simulink model "BattMPCv1"  (R2022b)
settings: Solver=VariableStepAuto  StartTime=0.0  StopTime=10.0  RelTol=1e-3
undefined symbols (not defined in the file): param
libraries: simulink x2, SOCMPC x1
settings Model: Creator=user  LastModifiedBy=user

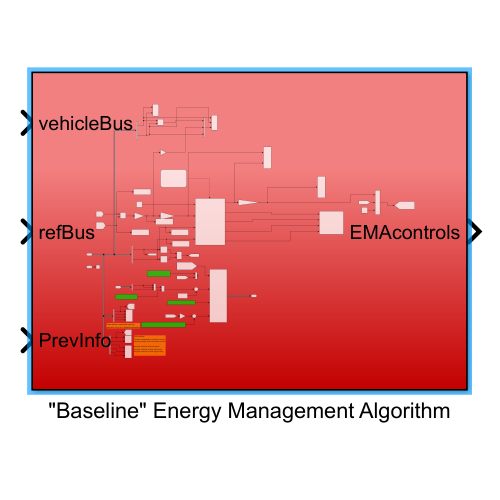
[thumbnail: Simulink's stored preview of the top-level diagram]
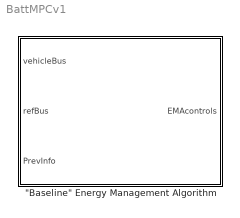
== system BattMPCv1 ==
  "\"Baseline\" Energy Management Algorithm" : Subsystem

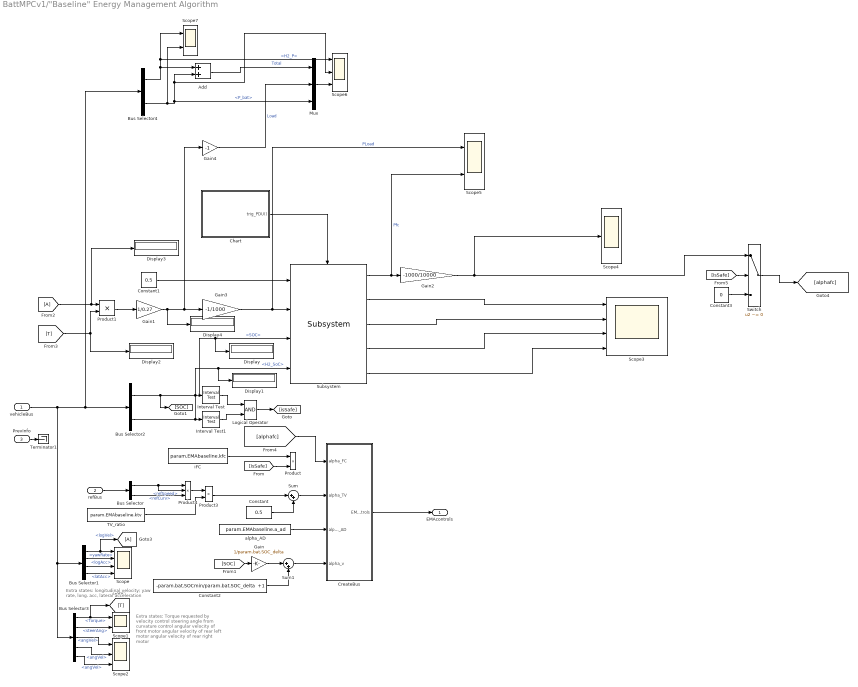
== system BattMPCv1/"Baseline" Energy Management Algorithm ==
  note: Extra states: longitudinal velocity;
      | yaw rate, long. acc, lateral acceleration
  note: Extra states:
      | Torque requested by velocity control
      | steering angle from curvature control
      |
      | angular velocity of front motor
      | angular velocity of rear left motor
      | angular velocity of rear right motor
  vehicleBus : Inport
  refBus : Inport  Port=2
  PrevInfo : Inport  Port=3
  Add : Sum
  Bus Selector : BusSelector  OutputSignals=refSpeed,refCurv
  Bus Selector1 : BusSelector  OutputSignals=chassisBus.logVel,chassisBus.yawRate,chassisBus.logAcc,chassisBus.latAcc
  Bus Selector2 : BusSelector  OutputSignals=batteryBus.SOC,rexBus.H2_SoC
  Bus Selector3 : BusSelector  OutputSignals=chassisControlBus.Torque,chassisControlBus.steerAng,electricMotorBusFM.angVel,electricMotorBusRL.angVel,electricMotorBusRR.angVel
  Bus Selector4 : BusSelector  OutputSignals=rexBus.H2_P,batteryBus.P_bat
  Chart : Stateflow chart  TreatAsAtomicUnit=on  SystemSampleTime=0.01
  Constant : Constant  Value=0.5
  Constant1 : Constant  Value=0.5
  Constant2 : Constant  Value="-param.bat.SOCmin/param.bat.SOC_delta  +1"
  Constant3 : Constant  Value=0
  CreateBus : Subsystem
  Display{,1..4} (5 alike) : Display
  From2 : From
  Gain : Gain  Gain=1/param.bat.SOC_delta
  Gain1 : Gain  Gain=1/0.27
  Gain2 : Gain  Gain=-1000/10000
  Gain3 : Gain  Gain=-1/1000
  Gain4 : Gain  Gain=-1
  Goto3 : Goto
  Interval Test : simulink/Logic and Bit Operations/Interval Test  IntervalClosedRight=on  uplimit=param.bat.SOCmax  IntervalClosedLeft=on  lowlimit=param.bat.SOCmin  OutDataTypeStr=boolean
  Interval Test1 : simulink/Logic and Bit Operations/Interval Test  IntervalClosedRight=on  uplimit=param.fuelcell.SOCmax  IntervalClosedLeft=on  lowlimit=param.fuelcell.SOCmin  OutDataTypeStr=boolean
  Logical Operator : Logic  AllPortsSameDT=off  OutDataTypeStr=boolean
  Mux : Mux  Inputs=3
  Product : Product
  Product1 : Product
  Product3 : Product
  Product4 : Product  Inputs=3
  Scope : Scope  NumInputPorts=4
  Scope1 : Scope  NumInputPorts=2
  Scope2 : Scope  NumInputPorts=3
  Scope3 : Scope  NumInputPorts=4
  Scope4 : Scope
  Scope5 : Scope  NumInputPorts=2
  Scope6 : Scope  NumInputPorts=3
  Scope7 : Scope  NumInputPorts=2
  Subsystem : SOCMPC/Subsystem  SystemSampleTime=-1  VariantActivationTime=update diagram  Latency=0  AutoFrameSizeCalculation=off
      link override Constrained: Gain=1
      link override Not Constrained: Gain=1
  Sum : Sum  Inputs=|++
  Sum1 : Sum  Inputs=|++
  Switch : Switch  Criteria=u2 ~= 0  SaturateOnIntegerOverflow=off  InputSameDT=off
  TV_ratio : Constant  Value=param.EMAbaseline.ktv
  Terminator1 : Terminator
  alpha_AD : Constant  Value=param.EMAbaseline.a_ad
  iFC : Constant  Value=param.EMAbaseline.kfc
  EMAcontrols : Outport
  wires:
  vehicleBus/1 -> Bus Selector4/1, Bus Selector2/1, Bus Selector3/1, Bus Selector1/1
  iFC/1 -> Product/1
  Bus Selector2/2 -> Display1/1, Subsystem/4, Interval Test1/1  "<H2_SoC>"
  Bus Selector2/1 -> [SOC], Display/1, Subsystem/3, Interval Test/1  "<SOC>"
  Interval Test/1 -> Logical Operator/1
  Interval Test1/1 -> Logical Operator/2
  CreateBus/1(EMAcontrols) -> EMAcontrols/1
  Logical Operator/1 -> [isSafe]
  [isSafe] -> Product/2
  TV_ratio/1 -> Product3/2
  Product4/1 -> Product3/1
  refBus/1 -> Bus Selector/1
  Bus Selector/2 -> Product4/3  "<refCurv>"
  Bus Selector/1 -> Product4/2, Product4/1  "<refSpeed>"
  Constant/1 -> Sum/2
  Product3/1 -> Sum/1
  [SOC] -> Gain/1
  Gain/1 -> Sum1/1
  Constant2/1 -> Sum1/2
  PrevInfo/1 -> Terminator1/1
  Sum/1 -> CreateBus/2(alpha_TV)
  alpha_AD/1 -> CreateBus/3(alpha_AD)
  Sum1/1 -> CreateBus/4(alpha_v)
  Bus Selector1/1 -> Goto3/1, Scope/1  "<logVel>"
  Bus Selector1/2 -> Scope/2  "<yawRate>"
  Bus Selector1/3 -> Scope/3  "<logAcc>"
  Bus Selector1/4 -> Scope/4  "<latAcc>"
  Bus Selector3/1 -> [T], Scope1/1  "<Torque>"
  Bus Selector3/2 -> Scope1/2  "<steerAng>"
  Bus Selector3/3 -> Scope2/1  "<angVel>"
  Bus Selector3/4 -> Scope2/2  "<angVel>"
  Bus Selector3/5 -> Scope2/3  "<angVel>"
  Constant1/1 -> Subsystem/1
  From2/1 -> Display3/1, Product1/1
  [T] -> Product1/2, Display2/1
  Product1/1 -> Gain1/1
  Gain1/1 -> Display4/1, Gain4/1, Gain3/1
  Subsystem/1 -> Scope5/2, Gain2/1  "Pfc"
  [alphafc] -> CreateBus/1(alpha_FC)
  Subsystem/2 -> Scope3/1
  Subsystem/3 -> Scope3/2
  Subsystem/4 -> Scope3/3
  Subsystem/5 -> Scope3/4
  Chart/1(trig_PDU()) -> Subsystem/Trigger
  Gain3/1 -> Scope5/1, Subsystem/2  "PLoad"
  Gain2/1 -> Switch/1, Scope4/1
  Bus Selector4/1 -> Scope7/1, Scope6/1, Add/1  "<H2_P>"
  Bus Selector4/2 -> Scope7/2, Mux/3, Scope6/2, Add/2  "<P_bat>"
  Mux/1 -> Scope6/3
  Add/1 -> Mux/1  "Total"
  Gain4/1 -> Mux/2  "Load"
  Switch/1 -> [alphafc]
  Constant3/1 -> Switch/3
  [isSafe] -> Switch/2

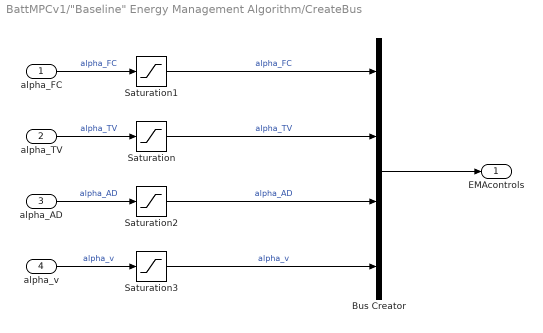
== system BattMPCv1/"Baseline" Energy Management Algorithm/CreateBus ==
  alpha_FC : Inport
  alpha_TV : Inport  Port=2
  alpha_AD : Inport  Port=3
  alpha_v : Inport  Port=4
  Bus Creator : BusCreator  Inputs=4
  Saturation{,1..3} (4 alike) : Saturate  UpperLimit=1  LowerLimit=0
  EMAcontrols : Outport
  wires:
  Saturation1/1 -> Bus Creator/1  "alpha_FC"
  Bus Creator/1 -> EMAcontrols/1
  Saturation/1 -> Bus Creator/2  "alpha_TV"
  Saturation2/1 -> Bus Creator/3  "alpha_AD"
  Saturation3/1 -> Bus Creator/4  "alpha_v"
  alpha_TV/1 -> Saturation/1  "alpha_TV"
  alpha_v/1 -> Saturation3/1  "alpha_v"
  alpha_AD/1 -> Saturation2/1  "alpha_AD"
  alpha_FC/1 -> Saturation1/1  "alpha_FC"

== stateflow chart BattMPCv1/"Baseline" Energy Management Algorithm/Chart ==
  (default) -> (junction 1)
  (junction 1) -> (junction 3) : {trig_PDU;}
  events: trig_PDU output FUNCTION_CALL_EVENT
